simulink library "ReceiveFromGES"  (R2016b)
settings: Solver=VariableStepAuto  StartTime=0.0  StopTime=10.0  RelTol=1e-3
libraries: ReceiveFromGES x3, simulink_extras x3, xpcethercatlib x1, VariousLibrary x1
settings Model: Creator=Nathan  LastModifiedBy=snyke7

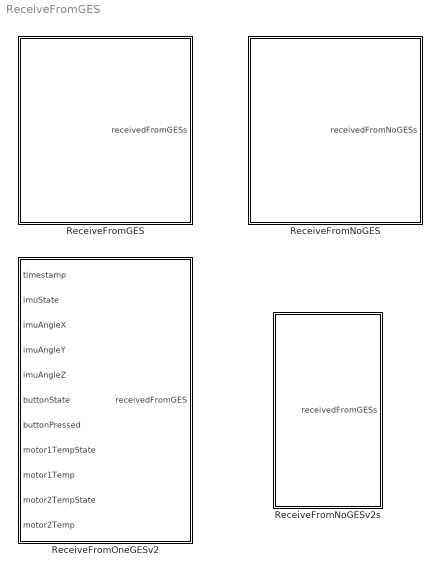
== system ReceiveFromGES ==
  ReceiveFromGES : Subsystem
  ReceiveFromNoGES : Subsystem
  ReceiveFromNoGESv2s : Subsystem
  ReceiveFromOneGESv2 : Subsystem

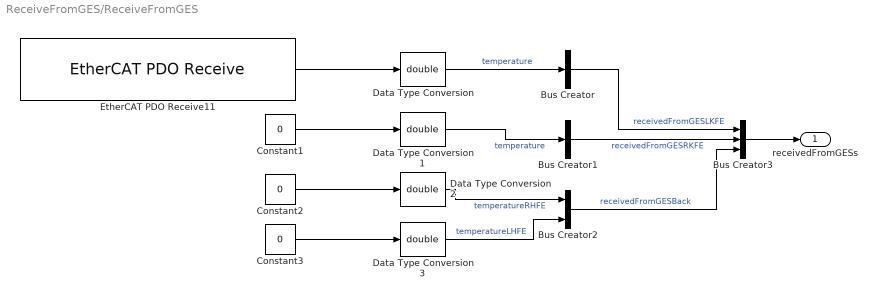
== system ReceiveFromGES/ReceiveFromGES ==
  Bus Creator : BusCreator  Inputs=1  OutDataTypeStr=Bus: EtherCATReceivedFromGESJoint  NonVirtualBus=on
  Bus Creator1 : BusCreator  Inputs=1  OutDataTypeStr=Bus: EtherCATReceivedFromGESJoint  NonVirtualBus=on
  Bus Creator2 : BusCreator  Inputs=2  OutDataTypeStr=Bus: EtherCATReceivedFromGESBack  NonVirtualBus=on
  Bus Creator3 : BusCreator  Inputs=3  OutDataTypeStr=Bus: EtherCATReceivedFromGES  NonVirtualBus=on
  Constant1 : Constant  Value=0
  Constant2 : Constant  Value=0
  Constant3 : Constant  Value=0
  Data Type Conversion{,1..3} (4 alike) : DataTypeConversion  OutDataTypeStr=double
  EtherCAT PDO Receive11 : xpcethercatlib/EtherCAT PDO Receive  Priority=2  sig_name=Box 2 (EasyCAT 32+32 configurable PDO).Inputs.temperature  sig_offset=728  sig_type=single  type_size=32  sig_dim=1  device_id=0  sample_time=0.002000
  receivedFromGESs : Outport  OutDataTypeStr=Bus: EtherCATReceivedFromGES
  wires:
  Data Type Conversion3/1 -> Bus Creator2/2  "temperatureLHFE"
  Bus Creator3/1 -> receivedFromGESs/1
  Bus Creator/1 -> Bus Creator3/1  "receivedFromGESLKFE"
  Bus Creator2/1 -> Bus Creator3/3  "receivedFromGESBack"
  Bus Creator1/1 -> Bus Creator3/2  "receivedFromGESRKFE"
  Data Type Conversion/1 -> Bus Creator/1  "temperature"
  Data Type Conversion2/1 -> Bus Creator2/1  "temperatureRHFE"
  Data Type Conversion1/1 -> Bus Creator1/1  "temperature"
  Constant1/1 -> Data Type Conversion1/1
  Constant2/1 -> Data Type Conversion2/1
  Constant3/1 -> Data Type Conversion3/1
  EtherCAT PDO Receive11/1 -> Data Type Conversion/1

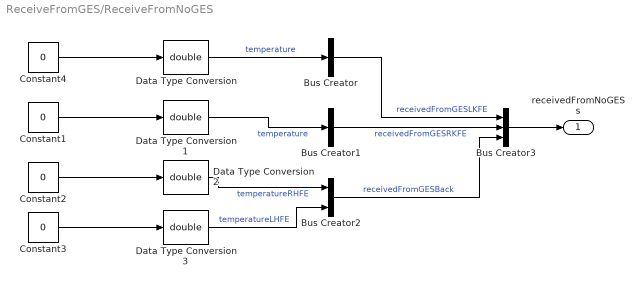
== system ReceiveFromGES/ReceiveFromNoGES ==
  Bus Creator : BusCreator  Inputs=1  OutDataTypeStr=Bus: EtherCATReceivedFromGESJoint  NonVirtualBus=on
  Bus Creator1 : BusCreator  Inputs=1  OutDataTypeStr=Bus: EtherCATReceivedFromGESJoint  NonVirtualBus=on
  Bus Creator2 : BusCreator  Inputs=2  OutDataTypeStr=Bus: EtherCATReceivedFromGESBack  NonVirtualBus=on
  Bus Creator3 : BusCreator  Inputs=3  OutDataTypeStr=Bus: EtherCATReceivedFromGES  NonVirtualBus=on
  Constant{1..4} (4 alike) : Constant  Value=0
  Data Type Conversion{,1..3} (4 alike) : DataTypeConversion  OutDataTypeStr=double
  receivedFromNoGESs : Outport  OutDataTypeStr=Bus: EtherCATReceivedFromGES
  wires:
  Constant4/1 -> Data Type Conversion/1
  Constant3/1 -> Data Type Conversion3/1
  Constant2/1 -> Data Type Conversion2/1
  Constant1/1 -> Data Type Conversion1/1
  Data Type Conversion1/1 -> Bus Creator1/1  "temperature"
  Data Type Conversion2/1 -> Bus Creator2/1  "temperatureRHFE"
  Data Type Conversion/1 -> Bus Creator/1  "temperature"
  Bus Creator1/1 -> Bus Creator3/2  "receivedFromGESRKFE"
  Bus Creator2/1 -> Bus Creator3/3  "receivedFromGESBack"
  Bus Creator/1 -> Bus Creator3/1  "receivedFromGESLKFE"
  Bus Creator3/1 -> receivedFromNoGESs/1
  Data Type Conversion3/1 -> Bus Creator2/2  "temperatureLHFE"

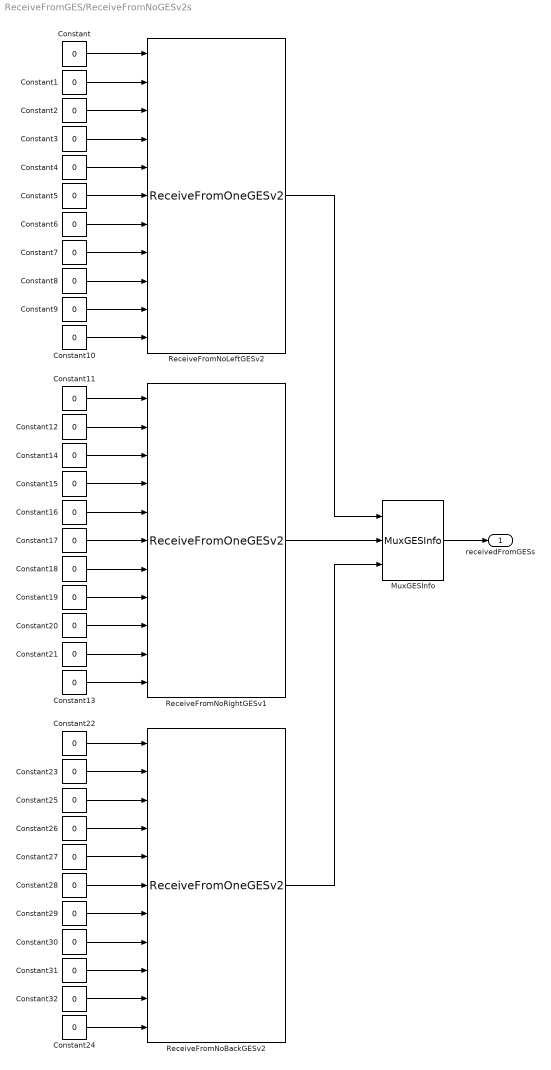
== system ReceiveFromGES/ReceiveFromNoGESv2s ==
  Constant{,1..32} (33 alike) : Constant  Value=0
  MuxGESInfo : VariousLibrary/MuxGESInfo
  ReceiveFromNoBackGESv2 : ReceiveFromGES/ReceiveFromOneGESv2
  ReceiveFromNoLeftGESv2 : ReceiveFromGES/ReceiveFromOneGESv2
  ReceiveFromNoRightGESv1 : ReceiveFromGES/ReceiveFromOneGESv2
  receivedFromGESs : Outport
  wires:
  Constant/1 -> ReceiveFromNoLeftGESv2/1
  Constant1/1 -> ReceiveFromNoLeftGESv2/2
  Constant4/1 -> ReceiveFromNoLeftGESv2/5
  Constant2/1 -> ReceiveFromNoLeftGESv2/3
  Constant5/1 -> ReceiveFromNoLeftGESv2/6
  Constant10/1 -> ReceiveFromNoLeftGESv2/11
  Constant7/1 -> ReceiveFromNoLeftGESv2/8
  Constant3/1 -> ReceiveFromNoLeftGESv2/4
  Constant6/1 -> ReceiveFromNoLeftGESv2/7
  Constant8/1 -> ReceiveFromNoLeftGESv2/9
  Constant9/1 -> ReceiveFromNoLeftGESv2/10
  Constant11/1 -> ReceiveFromNoRightGESv1/1
  Constant12/1 -> ReceiveFromNoRightGESv1/2
  Constant16/1 -> ReceiveFromNoRightGESv1/5
  Constant14/1 -> ReceiveFromNoRightGESv1/3
  Constant17/1 -> ReceiveFromNoRightGESv1/6
  Constant13/1 -> ReceiveFromNoRightGESv1/11
  Constant19/1 -> ReceiveFromNoRightGESv1/8
  Constant15/1 -> ReceiveFromNoRightGESv1/4
  Constant18/1 -> ReceiveFromNoRightGESv1/7
  Constant20/1 -> ReceiveFromNoRightGESv1/9
  Constant21/1 -> ReceiveFromNoRightGESv1/10
  Constant22/1 -> ReceiveFromNoBackGESv2/1
  Constant23/1 -> ReceiveFromNoBackGESv2/2
  Constant27/1 -> ReceiveFromNoBackGESv2/5
  Constant25/1 -> ReceiveFromNoBackGESv2/3
  Constant28/1 -> ReceiveFromNoBackGESv2/6
  Constant24/1 -> ReceiveFromNoBackGESv2/11
  Constant30/1 -> ReceiveFromNoBackGESv2/8
  Constant26/1 -> ReceiveFromNoBackGESv2/4
  Constant29/1 -> ReceiveFromNoBackGESv2/7
  Constant31/1 -> ReceiveFromNoBackGESv2/9
  Constant32/1 -> ReceiveFromNoBackGESv2/10
  ReceiveFromNoRightGESv1/1 -> MuxGESInfo/2
  ReceiveFromNoLeftGESv2/1 -> MuxGESInfo/1
  ReceiveFromNoBackGESv2/1 -> MuxGESInfo/3
  MuxGESInfo/1 -> receivedFromGESs/1

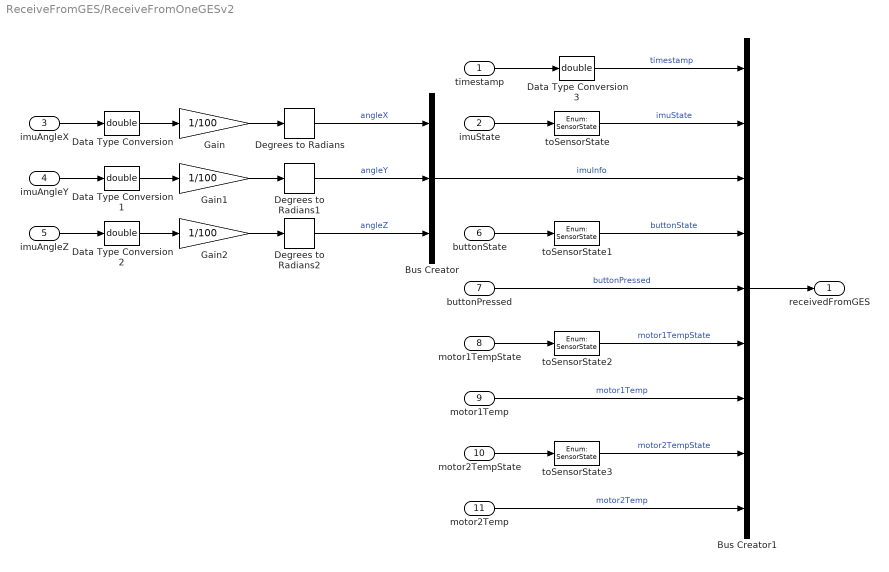
== system ReceiveFromGES/ReceiveFromOneGESv2 ==
  timestamp : Inport
  imuState : Inport  Port=2
  imuAngleX : Inport  Port=3
  imuAngleY : Inport  Port=4
  imuAngleZ : Inport  Port=5
  buttonState : Inport  Port=6
  buttonPressed : Inport  Port=7
  motor1TempState : Inport  Port=8
  motor1Temp : Inport  Port=9
  motor2TempState : Inport  Port=10
  motor2Temp : Inport  Port=11
  Bus Creator : BusCreator  Inputs=3  OutDataTypeStr=Bus: IMUInfo  NonVirtualBus=on
  Bus Creator1 : BusCreator  Inputs=9  OutDataTypeStr=Bus: EtherCATReceivedFromGES  NonVirtualBus=on
  Data Type Conversion{,1..3} (4 alike) : DataTypeConversion  OutDataTypeStr=double
  Degrees to Radians : simulink_extras/Transformations/Degrees to Radians
  Degrees to Radians1 : simulink_extras/Transformations/Degrees to Radians
  Degrees to Radians2 : simulink_extras/Transformations/Degrees to Radians
  Gain : Gain  Gain=1/100
  Gain1 : Gain  Gain=1/100
  Gain2 : Gain  Gain=1/100
  toSensorState{,1..3} (4 alike) : DataTypeConversion  OutDataTypeStr=Enum: SensorState  RndMeth=Nearest
  receivedFromGES : Outport
  wires:
  timestamp/1 -> Data Type Conversion3/1
  imuState/1 -> toSensorState/1
  Bus Creator/1 -> Bus Creator1/3  "imuInfo"
  motor2TempState/1 -> toSensorState3/1
  buttonPressed/1 -> Bus Creator1/5  "buttonPressed"
  motor1TempState/1 -> toSensorState2/1
  motor1Temp/1 -> Bus Creator1/7  "motor1Temp"
  motor2Temp/1 -> Bus Creator1/9  "motor2Temp"
  buttonState/1 -> toSensorState1/1
  Data Type Conversion/1 -> Gain/1
  imuAngleX/1 -> Data Type Conversion/1
  Degrees to Radians/1 -> Bus Creator/1  "angleX"
  imuAngleY/1 -> Data Type Conversion1/1
  Data Type Conversion1/1 -> Gain1/1
  Degrees to Radians1/1 -> Bus Creator/2  "angleY"
  imuAngleZ/1 -> Data Type Conversion2/1
  Data Type Conversion2/1 -> Gain2/1
  Degrees to Radians2/1 -> Bus Creator/3  "angleZ"
  Data Type Conversion3/1 -> Bus Creator1/1  "timestamp"
  Gain/1 -> Degrees to Radians/1
  Gain1/1 -> Degrees to Radians1/1
  Gain2/1 -> Degrees to Radians2/1
  toSensorState/1 -> Bus Creator1/2  "imuState"
  toSensorState1/1 -> Bus Creator1/4  "buttonState"
  toSensorState2/1 -> Bus Creator1/6  "motor1TempState"
  toSensorState3/1 -> Bus Creator1/8  "motor2TempState"
  Bus Creator1/1 -> receivedFromGES/1
